simulink model "restored"  (R2020a)
settings: Solver=ode1be  StartTime=0.0  StopTime=10  RelTol=1e-3
values from neighbouring files (symbols this model uses):
  c1 = 4.6210    (= 4.621)    [optimization_PID_SMC_Rotary_pendulum.m]
  c2 = 4.1349    [optimization_PID_SMC_Rotary_pendulum.m]
  Dp = 0.0005    [optimization_PID_SMC_Rotary_pendulum.m]
  Dr = 0.0015    [optimization_PID_SMC_Rotary_pendulum.m]
  g = 9.8    [optimization_PID_SMC_Rotary_pendulum.m]
  kd = 1.6452    [optimization_PID_SMC_Rotary_pendulum.m]
  ki = 1.9406    [optimization_PID_SMC_Rotary_pendulum.m]
  kp = 15.94461    [optimization_PID_SMC_Rotary_pendulum.m]
  Lp = 0.129    [optimization_PID_SMC_Rotary_pendulum.m]
  Lr = 0.085    [optimization_PID_SMC_Rotary_pendulum.m]
  mp = 0.024    [optimization_PID_SMC_Rotary_pendulum.m]
undefined symbols (not defined in the file or in its folder): hp, hr, mr
settings Model: Creator=user  LastModifiedBy=user
settings SolverCC: MaxConsecutiveMinStep=0.5  ConcurrentTasks=on
settings SFSimCC: SimAnalyzeCustomCode=on

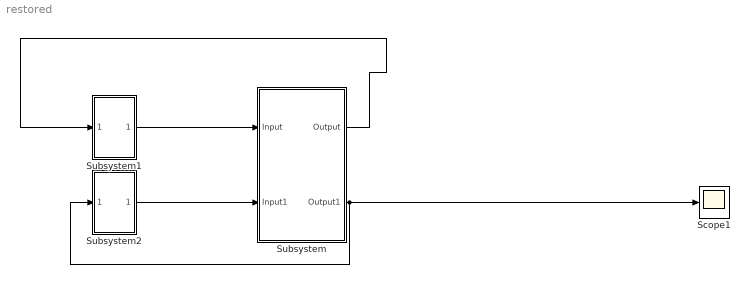
== system restored ==
  Scope1 : Scope
  Subsystem : Subsystem
  Subsystem1 : Subsystem
  Subsystem2 : Subsystem
  wires:
  Subsystem/1(Output) -> Subsystem1/1(Output1)
  Subsystem/2(Output1) -> Subsystem2/1(Output1), Scope1/1
  Subsystem1/1(Input) -> Subsystem/1(Input)
  Subsystem2/1(Input) -> Subsystem/2(Input1)

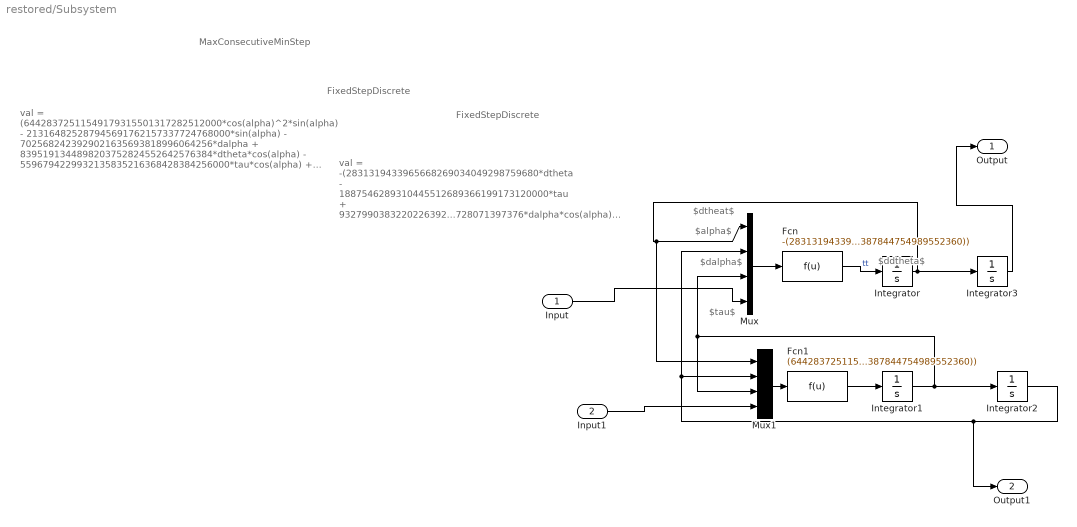
== system restored/Subsystem ==
  note: MaxConsecutiveMinStep
  note: FixedStepDiscrete
  note: FixedStepDiscrete
  note: val =
      |
      | (64428372511549179315501317282512000*cos(alpha)^2*sin(alpha) - 213164825287945691762157337724768000*sin(alpha) - 7025682423929021635693818996064256*dalpha + 8395191344898203752824552642576384*dtheta*cos(alpha) - 5596794229932135835216368428384256000*tau*cos(alpha) + 2123489575474251490005913125781504*dalpha*cos(alpha)^2 - 424043880305604253717562403602000*dtheta^2*cos(alpha)^3*sin(alpha) + 736426184774470493382792625276125*dalpha^2*cos(alpha)*sin(alpha) + 1402972574599234271768844492028000*dtheta^2*cos(alpha)*sin(alpha) + 1117635033363608135559535136403000*dalpha*dtheta*cos(alpha)^2*sin(alpha))/(375*(456091584978661951562070541663*cos(alpha)^2 + 4988346931908387844754989552360))
  note: $dalpha$
  note: $alpha$
  note: $tau$
  note: $dtheat$
  note: $ddtheta$
  note: val =
      |
      | -(2831319433965668269034049298759680*dtheta - 1887546289310445512689366199173120000*tau + 932799038322022639202728071397376*dalpha*cos(alpha) + 248363340747468440857360791163125*dalpha^2*sin(alpha) + 28301869061920828755811755676628000*cos(alpha)*sin(alpha) - 186272505560601355926589189400500*dtheta^2*cos(alpha)^2*sin(alpha) + 376927893604981507698010781435000*dalpha*dtheta*cos(alpha)*sin(alpha))/(125*(456091584978661951562070541663*cos(alpha)^2 + 4988346931908387844754989552360))
  Input : Inport
  Input1 : Inport  Port=2
  Fcn : Fcn  Expr=-(2831319433965668269034049298759680*u(1))-(1887546289310445512689366199173120000*u(4))+(932799038322022639202728071397376*u(3)*cos(u(2)))+(248363340747468440857360791163125*u(3)^2*sin(u(2)))+( 28301869061920828755811755676628000*cos(u(2))*sin(u(2)))-(186272505560601355926589189400500*u(1)^2*cos(u(2))^2*sin(u(2)))+(376927893604981507698010781435000*u(3)*u(1)*cos(u(2))*sin(u(2))) /(125*(456091584978661951562070541663*cos(u(3))^2 )+(4988346931908387844754989552360))
  Fcn1 : Fcn  Expr=(64428372511549179315501317282512000*cos(u(2))^2*sin(u(2))) -(213164825287945691762157337724768000*sin(u(2))-(7025682423929021635693818996064256*u(3))+(8395191344898203752824552642576384*u(1)*cos(u(2)) -(5596794229932135835216368428384256000*u(4))*cos(u(2)) +(2123489575474251490005913125781504*(u(3))*cos(u(2))^2 )-(424043880305604253717562403602000*u(3)^2*cos(u(2))^3*sin(u(2)))+(736426184774470493382792625276125*u(3)^2*cos(u(2))*sin(u(2))) +(1402972574599234271768844492028000*u(1)^2*cos(u(2))*sin(u(2)) )+(1117635033363608135559535136403000*u(3)*u(1))*cos(u(2))^2*sin(u(2)))/(375*(456091584978661951562070541663*cos(u(2))^2)) +( 4988346931908387844754989552360))
  Integrator{,1..3} (4 alike) : Integrator
  Mux : Mux
  Mux1 : Mux
  Output : Outport
  Output1 : Outport  Port=2
  wires:
  Integrator2/1 -> Mux1/2, Mux/2, Output1/1
  Mux1/1 -> Fcn1/1
  Integrator3/1 -> Output/1
  Fcn/1 -> Integrator/1  "tt"
  Fcn1/1 -> Integrator1/1
  Integrator/1 -> Integrator3/1, Mux1/1, Mux/1
  Input/1 -> Mux/4
  Mux/1 -> Fcn/1
  Integrator1/1 -> Integrator2/1, Mux1/3, Mux/3
  Input1/1 -> Mux1/4

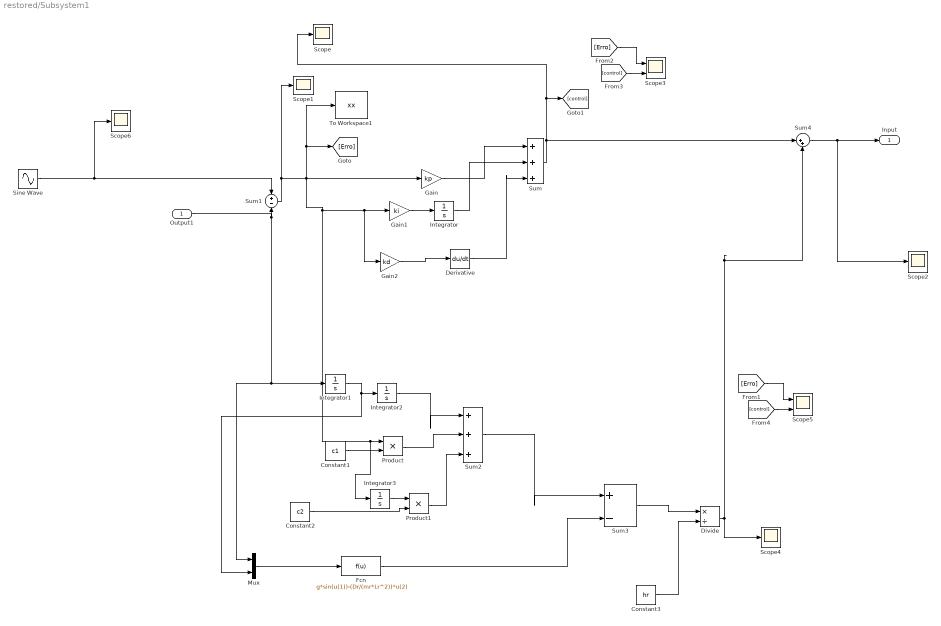
== system restored/Subsystem1 ==
  Output1 : Inport
  Constant1 : Constant  Value=c1
  Constant2 : Constant  Value=c2
  Constant3 : Constant  Value=hr
  Derivative : Derivative
  Divide : Product  Inputs=*/
  Fcn : Fcn  Expr=g*sin(u(1))-(Dr/(mr*Lr^2))*u(2)
  Gain : Gain  Gain=kp
  Gain1 : Gain  Gain=ki
  Gain2 : Gain  Gain=kd
  Integrator{,1..3} (4 alike) : Integrator
  Mux : Mux  Inputs=2
  Product : Product
  Product1 : Product
  Scope{,1..2,4,6} (5 alike) : Scope
  Scope3 : Scope  NumInputPorts=2
  Scope5 : Scope  NumInputPorts=2
  Sine Wave : Sin  Frequency=2  SampleTime=0
  Sum : Sum  Inputs=|+++
  Sum1 : Sum  Inputs=+-
  Sum2 : Sum  Inputs=|+++
  Sum3 : Sum  Inputs=|+-
  Sum4 : Sum  Inputs=|++
  To Workspace1 : ToWorkspace  VariableName=xx  SaveFormat=Structure With Time  SampleTime=-1
  Input : Outport
  wires:
  Sum/1 -> Sum4/1, [control], Scope/1
  Gain/1 -> Sum/1
  Gain1/1 -> Integrator/1
  Integrator/1 -> Sum/2
  Gain2/1 -> Derivative/1
  Derivative/1 -> Sum/3
  [Erro] -> Scope3/1
  [control] -> Scope3/2
  Integrator3/1 -> Product1/1
  Product1/1 -> Sum2/3
  Sum3/1 -> Divide/1
  Constant3/1 -> Divide/2
  Integrator2/1 -> Sum2/1
  Integrator1/1 -> Mux/2, Integrator2/1
  Sum1/1 -> Scope1/1, To Workspace1/1, [Erro], Integrator3/1, Product/1, Gain2/1, Gain1/1, Gain/1
  Product/1 -> Sum2/2
  Output1/1 -> Integrator1/1, Mux/1, Sum1/2
  Sum2/1 -> Sum3/1
  Fcn/1 -> Sum3/2
  [Erro] -> Scope5/1
  Divide/1 -> Sum4/2, Scope4/1
  [control] -> Scope5/2
  Constant1/1 -> Product/2
  Mux/1 -> Fcn/1
  Constant2/1 -> Product1/2
  Sum4/1 -> Scope2/1, Input/1
  Sine Wave/1 -> Scope6/1, Sum1/1

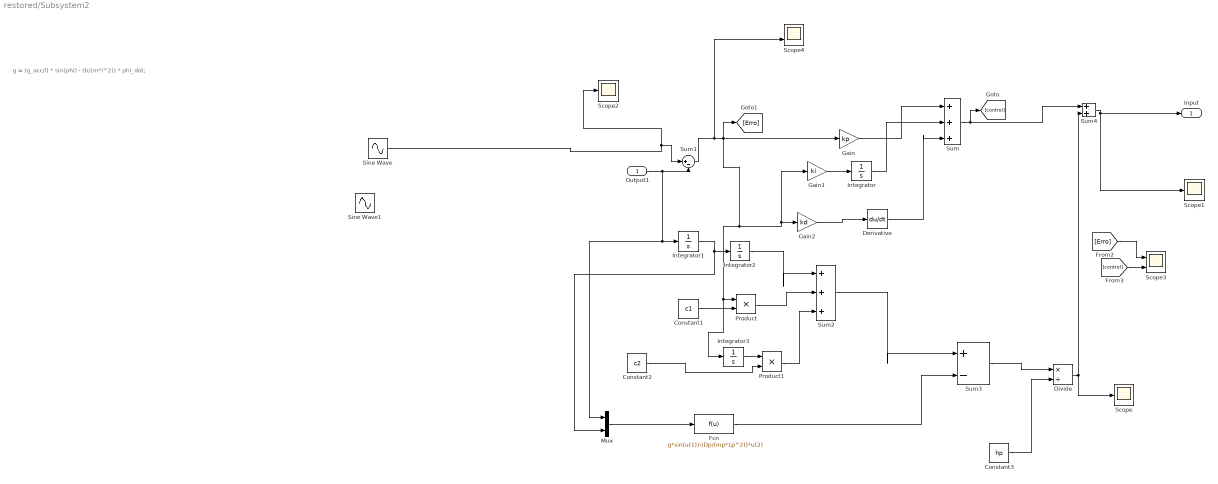
== system restored/Subsystem2 ==
  note: g = (g_acc/l) * sin(phi) - (b/(m*l^2)) * phi_dot;
  Output1 : Inport
  Constant1 : Constant  Value=c1
  Constant2 : Constant  Value=c2
  Constant3 : Constant  Value=hp
  Derivative : Derivative
  Divide : Product  Inputs=*/
  Fcn : Fcn  Expr=g*sin(u(1))-(Dp/(mp*Lp^2))*u(2)
  Gain : Gain  Gain=kp
  Gain1 : Gain  Gain=ki
  Gain2 : Gain  Gain=kd
  Integrator{,1..3} (4 alike) : Integrator
  Mux : Mux  Inputs=2
  Product : Product
  Product1 : Product
  Scope : Scope
  Scope1 : Scope
  Scope2 : Scope
  Scope3 : Scope  NumInputPorts=2
  Scope4 : Scope  NumInputPorts=2
  Sine Wave : Sin  Frequency=2  SampleTime=0
  Sine Wave1 : Sin  Frequency=2  SampleTime=0
  Sum : Sum  Inputs=|+++
  Sum1 : Sum  Inputs=|+-
  Sum2 : Sum  Inputs=|+++
  Sum3 : Sum  Inputs=|+-
  Sum4 : Sum  Inputs=|++
  Input : Outport
  wires:
  [Erro] -> Scope3/1
  [control] -> Scope3/2
  Gain1/1 -> Integrator/1
  Gain/1 -> Sum/1
  Sum1/1 -> Scope4/2, [Erro], Integrator3/1, Product/1, Gain1/1, Gain2/1, Gain/1
  Derivative/1 -> Sum/3
  Sum/1 -> Sum4/1, [control]
  Integrator/1 -> Sum/2
  Gain2/1 -> Derivative/1
  Integrator1/1 -> Mux/2, Integrator2/1
  Integrator2/1 -> Sum2/1
  Constant1/1 -> Product/2
  Product/1 -> Sum2/2
  Constant2/1 -> Product1/2
  Integrator3/1 -> Product1/1
  Product1/1 -> Sum2/3
  Sum2/1 -> Sum3/1
  Fcn/1 -> Sum3/2
  Sum3/1 -> Divide/1
  Constant3/1 -> Divide/2
  Divide/1 -> Sum4/2, Scope/1
  Sum4/1 -> Scope1/1, Input/1
  Mux/1 -> Fcn/1
  Output1/1 -> Mux/1, Integrator1/1, Sum1/2
  Sine Wave/1 -> Sum1/1, Scope2/1
